simulink model "FMU_Seperator_fmu"  (R2020b)
settings: Solver=VariableStepAuto  StartTime=0.0  StopTime=Inf  RelTol=1e-3
settings Model: Creator=kaebi  LastModifiedBy=kaebi

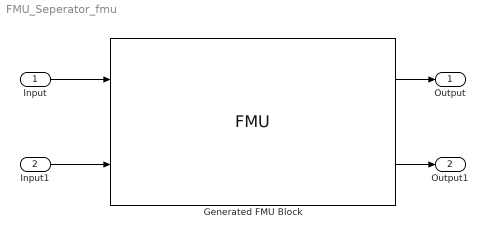
== system FMU_Seperator_fmu ==
  Input : Inport
  Input1 : Inport  Port=2
  Generated FMU Block : FMU  FMUName=FMU_Seperator  FMUMode=CoSimulation  FMUSampleTime=ts
      mask Type: FMU_Seperator [Co-Simulation, v2.0]
      mask Display:
      | if (exist([Simulink.fileGenControl('get','CacheFolder') '\slprj\_fmu\ec4a747b935d24d70922c4aa2f17c721\FMU_Seperator\model.png'],'file'))
      |     image([Simulink.fileGenControl('get','CacheFolder') '\slprj\_fmu\ec4a747b935d24d70922c4aa2f17c721\FMU_Seperator\model.png']);
      | else
      |     disp('FMU_Seperator');
      | end
      | port_label('output',1,'ModelToPLC');
      | port_label('output',2,'ModelToSignal');
      | port_label('input',1,'SignalToModel');
      | port_label('input',2,'PLCToModel');
  Output : Outport
  Output1 : Outport  Port=2
  wires:
  Input/1 -> Generated FMU Block/1
  Input1/1 -> Generated FMU Block/2
  Generated FMU Block/1 -> Output/1
  Generated FMU Block/2 -> Output1/1
